simulink subsystem "TransferCase"  (R2025b)
settings: Solver=VariableStepAuto  StartTime=0.0  StopTime=10.0  RelTol=1e-3
undefined symbols (not defined in the file): PlntDriveshftDamp, PlntDriveshftStiff
libraries: autolibsharedcoupling x2, autolibshareddiff x1
settings Model: Creator=The MathWorks, Inc.  LastModifiedBy=The MathWorks, Inc.
settings RTWCC: GPUComputeCapability=3.5

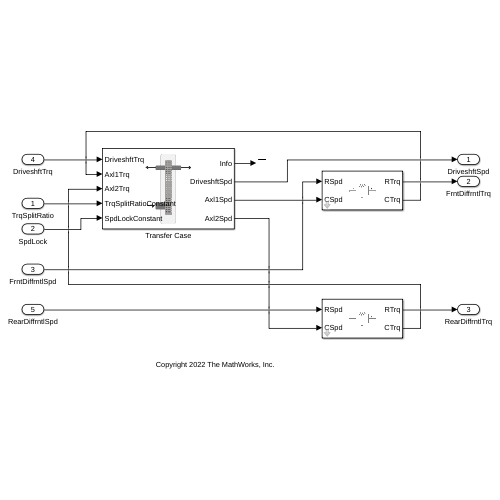
[thumbnail: Simulink's stored preview of the top-level diagram]
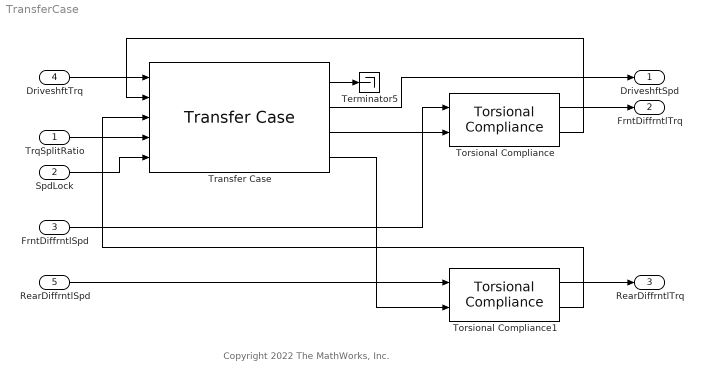
== system TransferCase ==
  note: Copyright 2022 The MathWorks, Inc.
  TrqSplitRatio : Inport
  SpdLock : Inport  Port=2
  FrntDiffrntlSpd : Inport  Port=3
  DriveshftTrq : Inport  Port=4
  RearDiffrntlSpd : Inport  Port=5
  Terminator5 : Terminator
  Torsional Compliance : autolibsharedcoupling/Torsional Compliance  port_config=Simulink  extInfo=off  k=PlntDriveshftStiff  b=PlntDriveshftDamp  theta_o=PlntDriveshftInitDeflect  domega_o=PlntDriveshftInitVel  omega_c=PlntDriveshftDampCutoffFreq  blkID=0  aMode=6
  Torsional Compliance1 : autolibsharedcoupling/Torsional Compliance  port_config=Simulink  extInfo=off  k=PlntDriveshftStiff  b=PlntDriveshftDamp  theta_o=PlntDriveshftInitDeflect  domega_o=PlntDriveshftInitVel  omega_c=PlntDriveshftDampCutoffFreq  blkID=0  aMode=6
  Transfer Case : autolibshareddiff/Transfer Case  DiffEffModelPopup=Constant  InterpMethod=Linear point-slope  extTamb=off  TrqSplitRatioMode=on  SpdLockMode=on  shaftSwitchMask=To the left of center-line  Ndiff=PlntTrnsfrCaseRatio  Jd=PlntTrnsfrCaseCarrInertia  bd=PlntTrnsfrCaseCarrDamp  Jw1=PlntTrnsfrCaseAxl1Inertia  bw1=PlntTrnsfrCaseAxl1Damp  Jw2=PlntTrnsfrCaseAxl2Inertia  bw2=PlntTrnsfrCaseAxl2Damp  omegaw1o=PlntTrnsfrCaseAxl1InitVel  omegaw2o=PlntTrnsfrCaseAxl2InitVel  eta=PlntTrnsfrCaseEff  eta_tbl=reshape([0.64 0.76 0.8 0.81 0.83 0.84 0.84 0.56 0.73 0.78 0.8 0.83 0.84 0.84 0.54 0.71 0.77 0.8 0.82 0.84 0.84 0.53 0.71 0.77 0.8 0.83 0.84 0.84 0.51 0.71 0.77 0.8 0.83 0.84 0.85 0.52 0.7 0.77 0.8 0.83 0.84 0.85 0.51 0.71 0.76 0.79 0.83 0.84 0.85 0.5 0.69 0.76 0.79 0.82 0.84 0.85 0.45 0.68 0.75 0.78 0.82 0.84 0.85 0.43 0.67 0.74 0.78 0.81 0.83 0.84 0.38 0.63 0.71 0.75 0.8 0.82 0.83 0.81 0.86 0.88 0.89 0.89 0.89 0.9 0.77 0.85 0.87 0.88 0.89 0.9 0.9 0.72 0.82 0.86 0.87 0.88 0.89 0.9 0.68 0.8 0.84 0.86 0.88 0.89 0.89 0.67 0.8 0.84 0.86 0.88 0.89 0.9 0.67 0.8 0.84 0.86 0.88 0.89 0.9 0.65 0.8 0.84 0.86 0.88 0.89 0.9 0.64 0.79 0.83 0.86 0.88 0.89 0.9 0.63 0.78 0.83 0.86 0.88 0.89 0.9 0.59 0.76 0.82 0.85 0.87 0.89 0.9 0.53 0.73 0.8 0.83 0.86 0.88 0.89], 7, 11, 2)  Trq_bpts=[25, 50, 75, 100, 150, 200, 250]  omega_bpts=[52.4 78.5 105 131 157 183 209 262 314 419 524]  Temp_bpts=[290 358]  Tamb=297.15  maxAbsSpd=5e3  aMode=6  TrqSplitRatio=0.5  SpdLock=0
      settings: LibrarySourceBlock=autolibdiff/Transfer Case
  DriveshftSpd : Outport
  FrntDiffrntlTrq : Outport  Port=2
  RearDiffrntlTrq : Outport  Port=3
  wires:
  SpdLock/1 -> Transfer Case/5
  TrqSplitRatio/1 -> Transfer Case/4
  Torsional Compliance1/2 -> Transfer Case/3
  Torsional Compliance1/1 -> RearDiffrntlTrq/1
  FrntDiffrntlSpd/1 -> Torsional Compliance/1
  Transfer Case/3 -> Torsional Compliance/2
  Transfer Case/1 -> Terminator5/1
  DriveshftTrq/1 -> Transfer Case/1
  RearDiffrntlSpd/1 -> Torsional Compliance1/1
  Torsional Compliance/1 -> FrntDiffrntlTrq/1
  Transfer Case/4 -> Torsional Compliance1/2
  Transfer Case/2 -> DriveshftSpd/1
  Torsional Compliance/2 -> Transfer Case/2
